simulink model "drm_simu"  (Simulink 8.6)
settings: Solver=VariableStepDiscrete  SolverMode=MultiTasking  StartTime=0.0  StopTime=12  RelTol=1e-3
PostLoadFcn:
  | init_drm
values from neighbouring files (symbols this model uses):
  sCRC_poly = struct(     'G16' ,{[1 0 0 0 1 0 0 0 0 0 0 1 0 0 0 0 1] ones(1,16)},     'G8'  ,{[1 0 0 0 1 1 1 0 1] ones(1,8)},     'G6'  ,{[1 1 0 1 1 1 1] ones(1,6)},     'G5'  ,{[1 1 0 1 1 1] ones(1,5)},     'G3'  ,{[1 0 1 0] ones(1,3)},     'G2'  ,{[1 1 1] ones(1,2)},     'G1'  ,{[1 1] 1} )    [crc_poly.m]
undefined symbols (not defined in the file or in its folder): channel, dfilt, fac, get, hot, if_mod, jet, magnitude, msc, ofdm, scrambler, sdc, sFFT, sync
libraries: dspmtrx3 x11, dspstat3 x7, commseqgen2 x6, dspobslib x6, dspsigops x5, commblkintrlv2 x4, dspsrcs4 x4, commsink2 x3, commrandsrc2 x3, commcrc2 x2, commcnvcod2 x2, commsequence2 x2
(part 2 of 2)

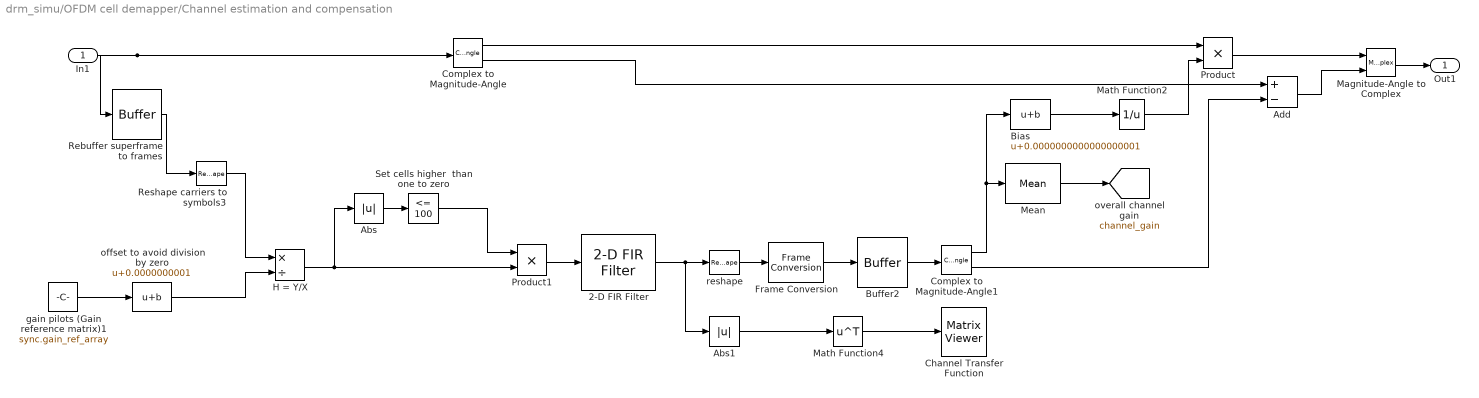
== system drm_simu/OFDM cell demapper/Channel estimation and compensation ==
  In1 : Inport
  2-D FIR Filter : visionfilter/2-D FIR Filter  separable=on  filtSrc=Specify via dialog  filterMtrx=[1 0; 0 -1]  verticalFilter=ones(1,channel.inter)  horizontalFilter=1  outSize=Same as input port I  padType=Circular  padSrc=Specify via dialog  padVal=1  method=Convolution  firstCoeffMode=Specify word length  firstCoeffWordLength=16  firstCoeffFracLength=0  firstCoeffSignedness=Signed  firstCoeffDataTypeStr=fixdt(1,16)  firstCoeffLastDataTypeStr=fixdt(1,16)  firstCoeffMin=[]  firstCoeffMax=[]  outputSignedness=Auto  outputMin=[]  outputMax=[]  accumDataTypeStr=Inherit: Same as product output  accumLastDataTypeStr=Inherit: Same as product output  prodOutputMode=Binary point scaling  prodOutputWordLength=32  prodOutputFracLength=10  prodOutputDataTypeStr=fixdt([],32,10)  prodOutputLastDataTypeStr=fixdt([],32,10)  roundingMode=Floor  overflowMode=off
  Abs : Abs
  Abs1 : Abs
  Add : Sum  Inputs=+-
  Bias : Bias  Bias=0.0000000000000000001
  Buffer2 : Buffer  N=ofdm.nmb_carriers*ofdm.nmb_symbols*3
  Channel Transfer Function : dspsnks4/Matrix Viewer  ImageParams=off  CMapStr=hot(256)  AxisColorbar=on  AxisParams=off  AxisOrigin=Upper left corner  XLabel=carrier k  YLabel=symbol s  ZLabel=|H_{est}|  FigPos=[351 349 991 420]  AxisZoom=off
      settings: YMin=0  YMax=2
  Complex to Magnitude-Angle : ComplexToMagnitudeAngle
  Complex to Magnitude-Angle1 : ComplexToMagnitudeAngle
  Frame Conversion : FrameConversion  InheritSamplingMode=off
  H = Y/X : Product  Inputs=*/
  Magnitude-Angle to Complex : MagnitudeAngleToComplex
  Math Function2 : Math  Operator=reciprocal  SaturateOnIntegerOverflow=on
  Math Function4 : Math  Operator=transpose  SaturateOnIntegerOverflow=on
  Mean : dspstat3/Mean  run=off  reset_popup=None  InputProcessing=Columns as channels (frame based)  directionMode=Each column  dimension=1  roiEnable=off  roiType=Rectangles  roiPortion=Entire ROI  roiOutput=Individual statistics for each ROI  roiFlag=off  outputDataTypeStr=Inherit: Same as accumulator  outputLastDataTypeStr=Inherit: Same as accumulator  outputMin=[]  outputMax=[]  roundingMode=Floor  overflowMode=off
  Product : Product  RndMeth=Zero
  Product1 : Product  RndMeth=Zero
  Rebuffer superframe to frames : Buffer  N=ofdm.nmb_carriers*ofdm.nmb_symbols
  Reshape carriers to symbols3 : Reshape  OutputDimensionality=Customize  OutputDimensions=[ofdm.nmb_carriers,ofdm.nmb_symbols]
  Set cells higher  than one to zero : simulink/Logic and Bit Operations/Compare To Constant  relop=<=  const=100  OutDataTypeStr=uint8  ZeroCross=off
  gain pilots (Gain reference matrix)1 : Constant  Value=sync.gain_ref_array  VectorParams1D=off
      settings: SamplingMode=Frame based
  offset to avoid division by zero : Bias  Bias=0.0000000001
  reshape : Reshape  OutputDimensionality=Column vector (2-D)  OutputDimensions=[ofdm.nmb_carriers,ofdm.nmb_symbols]
  Out1 : Outport
  tag scope: channel_gain=global
  wires:
  In1/1 -> Rebuffer superframe to frames/1, Complex to Magnitude-Angle/1
  Complex to Magnitude-Angle/1 -> Product/1
  Product/1 -> Magnitude-Angle to Complex/1
  Magnitude-Angle to Complex/1 -> Out1/1
  Rebuffer superframe to frames/1 -> Reshape carriers to symbols3/1
  Reshape carriers to symbols3/1 -> H = Y/X/1
  H = Y/X/1 -> Product1/2, Abs/1
  gain pilots (Gain reference matrix)1/1 -> offset to avoid division by zero/1
  offset to avoid division by zero/1 -> H = Y/X/2
  Set cells higher  than one to zero/1 -> Product1/1
  Product1/1 -> 2-D FIR Filter/1
  Math Function4/1 -> Channel Transfer Function/1
  2-D FIR Filter/1 -> reshape/1, Abs1/1
  reshape/1 -> Frame Conversion/1
  Buffer2/1 -> Complex to Magnitude-Angle1/1
  Frame Conversion/1 -> Buffer2/1
  Complex to Magnitude-Angle1/1 -> Bias/1, Mean/1
  Bias/1 -> Math Function2/1
  Math Function2/1 -> Product/2
  Abs1/1 -> Math Function4/1
  Add/1 -> Magnitude-Angle to Complex/2
  Complex to Magnitude-Angle1/2 -> Add/2
  Complex to Magnitude-Angle/2 -> Add/1
  Abs/1 -> Set cells higher  than one to zero/1
  Mean/1 -> [channel_gain]

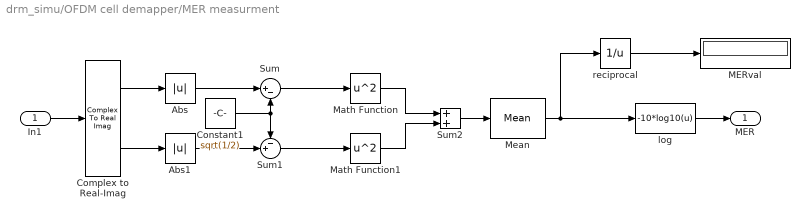
== system drm_simu/OFDM cell demapper/MER measurment ==
  In1 : Inport
  Abs : Abs
  Abs1 : Abs
  Complex to Real-Imag : ComplexToRealImag
  Constant1 : Constant  Value=sqrt(1/2)  SampleTime=-1  FramePeriod=65
  MERval : Display
  Math Function : Math  Operator=square  SaturateOnIntegerOverflow=on
  Math Function1 : Math  Operator=square  SaturateOnIntegerOverflow=on
  Mean : dspstat3/Mean  run=off  reset_popup=None  InputProcessing=Columns as channels (frame based)  directionMode=Each column  dimension=1  roiEnable=off  roiType=Rectangles  roiPortion=Entire ROI  roiOutput=Individual statistics for each ROI  roiFlag=off  outputDataTypeStr=Inherit: Same as accumulator  outputLastDataTypeStr=Inherit: Same as accumulator  outputMin=[]  outputMax=[]  roundingMode=Floor  overflowMode=off
  Sum : Sum  Inputs=|+-
  Sum1 : Sum  Inputs=-+|
  Sum2 : Sum
  log : Fcn  Expr=-10*log10(u)
  reciprocal : Math  Operator=reciprocal  SaturateOnIntegerOverflow=on
  MER : Outport
  wires:
  Complex to Real-Imag/1 -> Abs/1
  Complex to Real-Imag/2 -> Abs1/1
  Abs/1 -> Sum/1
  Abs1/1 -> Sum1/2
  Constant1/1 -> Sum/2, Sum1/1
  Sum/1 -> Math Function/1
  Sum1/1 -> Math Function1/1
  Math Function1/1 -> Sum2/2
  Math Function/1 -> Sum2/1
  Sum2/1 -> Mean/1
  Mean/1 -> log/1, reciprocal/1
  log/1 -> MER/1
  reciprocal/1 -> MERval/1
  In1/1 -> Complex to Real-Imag/1

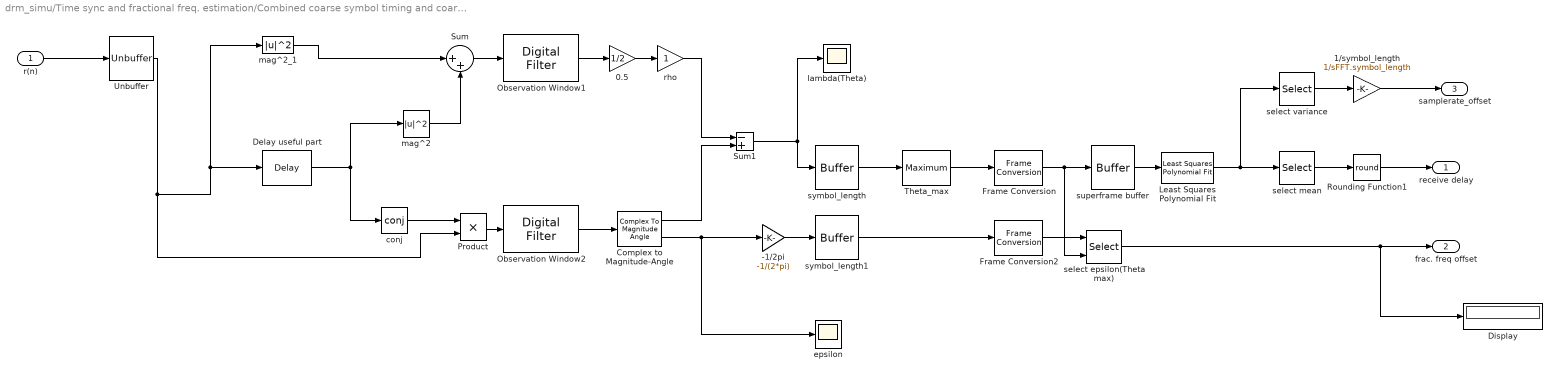
== system drm_simu/Time sync and fractional freq. estimation/Combined coarse symbol timing and coarse fractional frequency offset ==
  r(n) : Inport
  -1/2pi : Gain  Gain=-1/(2*pi)
  0.5 : Gain  Gain=1/2
  1/symbol_length : Gain  Gain=1/sFFT.symbol_length
  Complex to Magnitude-Angle : ComplexToMagnitudeAngle
  Delay useful part : dspobslib/Delay  InputProcessing=Inherited (this choice will be removed - see release notes)  dly_unit=Samples  delay=sFFT.size  ic_detail=off  dif_ic_for_ch=off  dif_ic_for_dly=off  ic=0  reset_popup=None
  Display : Display
  Frame Conversion : FrameConversion  InheritSamplingMode=off  OutFrame=Sample-based
  Frame Conversion2 : FrameConversion  InheritSamplingMode=off  OutFrame=Sample-based
  Least Squares Polynomial Fit : dsppolyfun/Least Squares Polynomial Fit  X=[0:ofdm.nmb_symbols*ofdm.superframe_size-1]  N=1
  Observation Window1 : dspobslib/Digital Filter  TypePopup=FIR (all zeros)  IIRFiltStruct=Direct form II transposed  AllPoleFiltStruct=Direct form  FIRFiltStruct=Direct form  CoeffSource=Specify via dialog  NumCoeffs=[ones(1,sFFT.guard_size)]  DenCoeffs=[1 0.1]  BiQuadCoeffs=[1 0.3 0.4 1 0.1 0.2]  LatticeCoeffs=[0.2 0.4]  denIgnore=on  FiltPerSampPopup=One filter per frame  IC=0  ICnum=0  ICden=0  roundingMode=Floor  overflowMode=off  ScaleValues=1  scaleValueFracLength=14  stageInFracLength=15  stageOutFracLength=15  FilterSource=Specify via dialog  dfiltObjectName=dfilt.dffir([1 2 1])  InputProcessing=Inherited (this choice will be removed - see release notes)
  Observation Window2 : dspobslib/Digital Filter  TypePopup=FIR (all zeros)  IIRFiltStruct=Direct form II transposed  AllPoleFiltStruct=Direct form  FIRFiltStruct=Direct form  CoeffSource=Specify via dialog  NumCoeffs=[ones(1,sFFT.guard_size)]  DenCoeffs=[1 0.1]  BiQuadCoeffs=[1 0.3 0.4 1 0.1 0.2]  LatticeCoeffs=[0.2 0.4]  denIgnore=on  FiltPerSampPopup=One filter per frame  IC=0  ICnum=0  ICden=0  roundingMode=Floor  overflowMode=off  ScaleValues=1  scaleValueFracLength=14  stageInFracLength=15  stageOutFracLength=15  FilterSource=Specify via dialog  dfiltObjectName=dfilt.dffir([1 2 1])  InputProcessing=Inherited (this choice will be removed - see release notes)
  Product : Product  RndMeth=Zero
  Rounding Function1 : Rounding  Operator=round
  Sum : Sum  Inputs=|++
  Sum1 : Sum  Inputs=-+
  Theta_max : dspstat3/Maximum  fcn=Index  reset=None  InputProcessing=Columns as channels (frame based)  indexBase=One  operateOver=Each column  Dimension=1  operation=maximum  roiEnable=off  roiType=Rectangles  roiPortion=Entire ROI  roiOutput=Individual statistics for each ROI  roiFlag=off  accumDataTypeStr=Inherit: Same as product output  accumLastDataTypeStr=Inherit: Same as product output  roundingMode=Floor  overflowMode=off
  Unbuffer : Unbuffer
  conj : Math  Operator=conj  SaturateOnIntegerOverflow=on
  epsilon : Scope
  lambda(Theta) : Scope
  mag^2 : Math  Operator=magnitude^2  SaturateOnIntegerOverflow=on
  mag^2_1 : Math  Operator=magnitude^2  SaturateOnIntegerOverflow=on
  rho : Gain
  select epsilon(Theta max) : Selector  InputPortWidth=sFFT.symbol_length  IndexOptions=Index vector (port)  Indices=[1 3]  OutputSizes=1
  select mean : Selector  InputPortWidth=2  IndexOptions=Index vector (dialog)  Indices=[2]  OutputSizes=1
  select variance : Selector  InputPortWidth=2  IndexOptions=Index vector (dialog)  Indices=[1]  OutputSizes=1
  superframe buffer : Buffer  N=ofdm.nmb_symbols*ofdm.superframe_size
  symbol_length : Buffer  N=sFFT.symbol_length
  symbol_length1 : Buffer  N=sFFT.symbol_length
  receive delay : Outport
  frac. freq offset : Outport  Port=2
  samplerate_offset : Outport  Port=3
  wires:
  Delay useful part/1 -> conj/1, mag^2/1
  mag^2/1 -> Sum/2
  mag^2_1/1 -> Sum/1
  Complex to Magnitude-Angle/1 -> Sum1/2
  Sum1/1 -> symbol_length/1, lambda(Theta)/1
  conj/1 -> Product/1
  Product/1 -> Observation Window2/1
  Sum/1 -> Observation Window1/1
  Observation Window2/1 -> Complex to Magnitude-Angle/1
  Unbuffer/1 -> mag^2_1/1, Delay useful part/1, Product/2
  Observation Window1/1 -> 0.5/1
  symbol_length/1 -> Theta_max/1
  Complex to Magnitude-Angle/2 -> epsilon/1, -1/2pi/1
  symbol_length1/1 -> Frame Conversion2/1
  select epsilon(Theta max)/1 -> frac. freq offset/1, Display/1
  -1/2pi/1 -> symbol_length1/1
  r(n)/1 -> Unbuffer/1
  0.5/1 -> rho/1
  Least Squares Polynomial Fit/1 -> select mean/1, select variance/1
  Rounding Function1/1 -> receive delay/1
  select mean/1 -> Rounding Function1/1
  select variance/1 -> 1/symbol_length/1
  1/symbol_length/1 -> samplerate_offset/1
  Frame Conversion2/1 -> select epsilon(Theta max)/1
  rho/1 -> Sum1/1
  superframe buffer/1 -> Least Squares Polynomial Fit/1
  Frame Conversion/1 -> superframe buffer/1, select epsilon(Theta max)/2
  Theta_max/1 -> Frame Conversion/1

== system drm_simu/demodulator/Downsampling ==
  In1 : Inport
  Decimation Filter : dsparch4/Digital Filter Design  mwdsp_browser_bugfix_var=off
  Downsample : DownSample  N=if_mod.upsample_factor  InputProcessing=Inherited (this choice will be removed - see release notes)  fmode=Maintain input frame rate
  Out1 : Outport
  wires:
  Decimation Filter/1 -> Downsample/1
  Downsample/1 -> Out1/1
  In1/1 -> Decimation Filter/1

== system drm_simu/demodulator/IF Demodulator ==
  s^(t) : Inport
  Cosine Wave : dspsrcs4/Sine Wave  Amplitude=1  Frequency=if_mod.if_freq  Phase=pi/2  SampleMode=Discrete  OutComplex=Real  CompMethod=Trigonometric fcn  TableSize=Speed  SampleTime=if_mod.sample_time  SamplesPerFrame=if_mod.frame_size  ResetState=Restart at time zero  OutputFrames=on  dataType=double  wordLen=16  udDataType=sfix(16)  fracBitsMode=Best precision  numFracBits=15  OutDataTypeStr=double  LastOutDataTypeStr=double
  InPhase Mixing Gain : Gain  Gain=sqrt(2)
  Product1 : Product  RndMeth=Zero
  Product2 : Product  RndMeth=Zero
  Quad Mixing Gain : Gain  Gain=sqrt(2)
  Real-Imag to Complex : RealImagToComplex
  Sine Wave : dspsrcs4/Sine Wave  Amplitude=1  Frequency=if_mod.if_freq  Phase=0  SampleMode=Discrete  OutComplex=Real  CompMethod=Trigonometric fcn  TableSize=Speed  SampleTime=if_mod.sample_time  SamplesPerFrame=if_mod.frame_size  ResetState=Restart at time zero  OutputFrames=on  dataType=double  wordLen=16  udDataType=sfix(16)  fracBitsMode=Best precision  numFracBits=15  OutDataTypeStr=double  LastOutDataTypeStr=double
  g^(t) : Outport
  wires:
  s^(t)/1 -> Product1/2, Product2/1
  Sine Wave/1 -> Product1/1
  Cosine Wave/1 -> Product2/2
  Product1/1 -> InPhase Mixing Gain/1
  Product2/1 -> Quad Mixing Gain/1
  Real-Imag to Complex/1 -> g^(t)/1
  Quad Mixing Gain/1 -> Real-Imag to Complex/2
  InPhase Mixing Gain/1 -> Real-Imag to Complex/1

== system drm_simu/modulator/IF Modulator ==
  s_b(t) : Inport
  Add : Sum
  Complex to Real-Imag : ComplexToRealImag
  Cosine Wave : dspsrcs4/Sine Wave  Amplitude=1  Frequency=if_mod.if_freq  Phase=0  SampleMode=Discrete  OutComplex=Real  CompMethod=Trigonometric fcn  TableSize=Speed  SampleTime=if_mod.sample_time  SamplesPerFrame=if_mod.frame_size  ResetState=Restart at time zero  OutputFrames=on  dataType=double  wordLen=16  udDataType=sfix(16)  fracBitsMode=Best precision  numFracBits=15  OutDataTypeStr=double  LastOutDataTypeStr=double
  InPhase Mixing Gain : Gain  Gain=sqrt(2)
  Product : Product  RndMeth=Zero
  Product2 : Product  RndMeth=Zero
  Quad Mixing Gain : Gain  Gain=sqrt(2)
  Sine Wave : dspsrcs4/Sine Wave  Amplitude=1  Frequency=if_mod.if_freq  Phase=pi/2  SampleMode=Discrete  OutComplex=Real  CompMethod=Trigonometric fcn  TableSize=Speed  SampleTime=if_mod.sample_time  SamplesPerFrame=if_mod.frame_size  ResetState=Restart at time zero  OutputFrames=on  dataType=double  wordLen=16  udDataType=sfix(16)  fracBitsMode=Best precision  numFracBits=15  OutDataTypeStr=double  LastOutDataTypeStr=double
  s(t) : Outport
  wires:
  Cosine Wave/1 -> Product/1
  Add/1 -> s(t)/1
  Product/1 -> InPhase Mixing Gain/1
  Product2/1 -> Quad Mixing Gain/1
  s_b(t)/1 -> Complex to Real-Imag/1
  Complex to Real-Imag/1 -> Product/2
  Complex to Real-Imag/2 -> Product2/1
  Sine Wave/1 -> Product2/2
  InPhase Mixing Gain/1 -> Add/1
  Quad Mixing Gain/1 -> Add/2

== system drm_simu/modulator/Upsampling ==
  In1 : Inport
  Gain : Gain  Gain=4
  Interpolation Filter : dsparch4/Digital Filter Design  mwdsp_browser_bugfix_var=off
  Upsample1 : dspsigops/Upsample  N=if_mod.upsample_factor  phase=0  InputProcessing=Inherited (this choice will be removed - see release notes)  RateOptions=Enforce single-rate processing  ic=0  mode=Unused parameter value
  Out1 : Outport
  wires:
  Upsample1/1 -> Interpolation Filter/1
  Interpolation Filter/1 -> Gain/1
  Gain/1 -> Out1/1
  In1/1 -> Upsample1/1
